simulink model "verify_Thermal_Node_mdl"  (R2016b)
settings: Solver=ode45  StartTime=0.0  StopTime=2*3600  MaxStep=100  RelTol=1e-3  EnableMultiTasking=on
libraries: simulink x1, carnot x1
settings Model: Creator=drhf  LastModifiedBy=srrt
settings DataIOCC: LimitDataPoints=on  SaveFormat=Array  SignalLoggingSaveFormat=ModelDataLogs
settings OptimizationCC: ExpressionDepthLimit=2147483647  LifeSpan=inf
settings DebuggingCC: UnderspecifiedInitializationDetection=Classic  MergeDetectMultiDrivingBlocksExec=none  SolverPrmCheckMsg=warning  FcnCallInpInsideContextMsg=warning  StateNameClashWarn=warning  SFUnexpectedBacktrackingDiag=warning  SFNoUnconditionalDefaultTransitionDiag=warning  SFExecutionAtInitializationDiag=none
settings HardwareCC: ProdBitPerPointer=32  ProdBitPerSizeT=32  ProdBitPerPtrDiffT=32  ProdLargestAtomicFloat=None  ProdIntDivRoundTo=Undefined  ProdEndianess=Unspecified  ProdWordSize=32  ProdHWDeviceType=32-bit Generic
settings ModelReferenceCC: PropagateSignalLabelsOutOfModel=off
settings GRTTargetCC: TargetLangStandard=C89/C90 (ANSI)  GeneratePreprocessorConditionals=Disable all  CombineOutputUpdateFcns=off  GRTInterface=on
settings ConfigComp: CovMetricSettings=dw  CovHtmlReporting=on  CovSaveCumulativeToWorkspaceVar=on  CovSaveSingleToWorkspaceVar=on  CovExternalEMLEnable=off

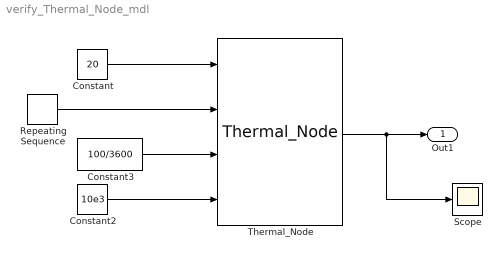
== system verify_Thermal_Node_mdl ==
  Constant : Constant  Value=20
  Constant2 : Constant  Value=10e3
  Constant3 : Constant  Value=100/3600
  Repeating Sequence : simulink/Sources/Repeating Sequence  rep_seq_t=[0 1 1.1 2]*3600  rep_seq_y=[15 15 25 25]
  Scope : Scope
  Thermal_Node : carnot/Basic/Thermal_Models/Thermal_Node  UA=1  mcp=10*4182  cp_approx=4182  Tini=20
  Out1 : Outport
  wires:
  Thermal_Node/1 -> Scope/1, Out1/1
  Repeating Sequence/1 -> Thermal_Node/2
  Constant/1 -> Thermal_Node/1
  Constant3/1 -> Thermal_Node/3
  Constant2/1 -> Thermal_Node/4
